simulink model "design_project_openloop_nonlinear"  (R2023b)
settings: Solver=FixedStepAuto  StartTime=0.0  StopTime=500  FixedStep=0.01  RelTol=1e-3
values from neighbouring files (symbols this model uses):
  delta_x_0 = 0    [design_project.m]
  delta_y_0 = 0    [design_project.m]
  x_0 = [1; 1; 1; 1]    [design_project.m]
settings Model: Creator=qingyu  LastModifiedBy=qingyu

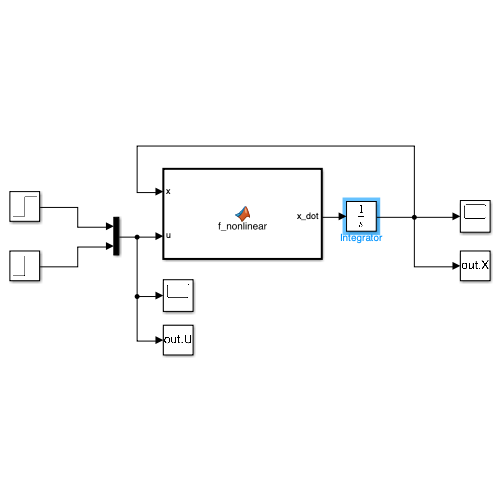
[thumbnail: Simulink's stored preview of the top-level diagram]
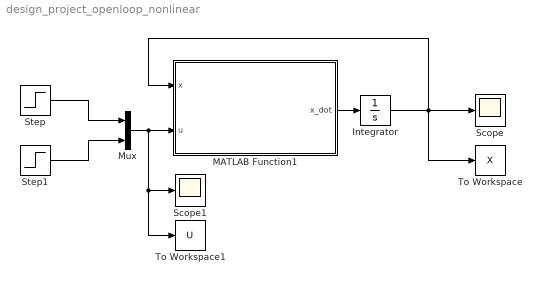
== system design_project_openloop_nonlinear ==
  Integrator : Integrator  InitialCondition=x_0
  MATLAB Function1 : MATLAB Function  TreatAsAtomicUnit=on
  Mux : Mux  Inputs=2
  Scope : Scope
  Scope1 : Scope
  Step : Step  After=delta_x_0  SampleTime=0
  Step1 : Step  After=delta_y_0  SampleTime=0
  To Workspace : ToWorkspace  VariableName=X  SampleTime=0.01
  To Workspace1 : ToWorkspace  VariableName=U  SampleTime=0.01
  wires:
  MATLAB Function1/1(x_dot) -> Integrator/1
  Integrator/1 -> To Workspace/1, Scope/1, MATLAB Function1/1(x)
  Step/1 -> Mux/1
  Step1/1 -> Mux/2
  Mux/1 -> Scope1/1, To Workspace1/1, MATLAB Function1/2(u)

== matlab function design_project_openloop_nonlinear/MATLAB Function1 ==
  data: x input; x_dot output; u input
function x_dot = f_nonlinear(x,u)

g               =  9.81;
v               =  350.3552;
m               =  320;
P               =  20000;
alpha           =  0.2618;
theta           = -0.0688;
vartheta        =  0.1930;
Z_delta_y       = -2018.0457;
Z_beta          =  13273.1810;

J_x             =  2.601;
J_y             =  751.8960;

M_x_omega_x     = -4.8379;
M_x_omega_y     = -1.7167;
M_x_beta        = -22.8888;
M_x_delta_x     = -2.5490;
M_x_delta_y     = -2.0289;

M_y_omega_x     = -15.0379;
M_y_omega_y     = -150.3792;
M_y_beta        = -2255.6880;
M_y_beta_dot    =  0;
M_y_delta_y     = -676.7064;

omega_z = 0;

omega_x = x(1);
omega_y = x(2);
beta    = x(3);
gamma   = x(4);

delta_x = u(1);
delta_y = u(2);

omega_x_dot = 0;
omega_x_dot = omega_x_dot + M_x_omega_x/J_x*omega_x;
omega_x_dot = omega_x_dot + M_x_omega_y/J_x*omega_y;
omega_x_dot = omega_x_dot + M_x_beta/J_x*beta;
omega_x_dot = omega_x_dot + M_x_delta_x/J_x*delta_x;
omega_x_dot = omega_x_dot + M_x_delta_y/J_x*delta_y;

gamma_dot = 0;
gamma_dot = gamma_dot + omega_x;
gamma_dot = gamma_dot - tand(vartheta)*(omega_y*cosd(gamma)-omega_z*sind(gamma));

beta_dot = 0;
beta_dot = beta_dot + cosd(theta)*(cosd(gamma)-omega_z*sind(gamma))/cosd(vartheta)*omega_y;
beta_dot = beta_dot - (P-Z_beta)/(m*v)*beta;
beta_dot = beta_dot + (g/v)*cosd(alpha)*sind(beta)*sind(vartheta);
beta_dot = beta_dot - (g/v)*sind(alpha)*sind(beta)*cosd(gamma)*cosd(vartheta);
beta_dot = beta_dot + (g/v)*cosd(beta)*sind(gamma)*cosd(vartheta);
beta_dot = beta_dot + alpha*gamma_dot;
beta_dot = beta_dot + Z_delta_y/(m*v)*delta_y;

omega_y_dot = 0;
omega_y_dot = omega_y_dot + M_y_omega_x/J_y*omega_x;
omega_y_dot = omega_y_dot + M_y_omega_y/J_y*omega_y;
omega_y_dot = omega_y_dot + M_y_beta/J_y*beta;
omega_y_dot = omega_y_dot + M_y_beta_dot/J_y*beta_dot;
omega_y_dot = omega_y_dot + M_y_delta_y/J_y*delta_y;

x_dot = [
    omega_x_dot;
    omega_y_dot;
    beta_dot;
    gamma_dot
];
